simulink model "sim_models"  (R2018b)
settings: Solver=FixedStepAuto  StartTime=0.0  StopTime=10  RelTol=1e-3
values from neighbouring files (symbols this model uses):
  Ts = 0.1    [KinematicBicycleModel.m]    (also in LeftLaneChangeSinusoidalMotionModel.m; LinearizedBicycleModel.m; SimplifiedKinematicBicycleModel.m; amm_rel_test.m)
  vx = X(2)    [cv_model_fun.m]    (also in initialization.m = 10)
  vy = X(4)    [cv_model_fun.m]    (also in initialization.m = 0)
  x = X(1)    [KinematicBicycleModel.m]    (also in SimplifiedKinematicBicycleModel.m; behavior_model.m = 0:0.01:20; cca_model_fun.m; ctra_model_fun.m)
  y = X(2)    [KinematicBicycleModel.m]    (also in SimplifiedKinematicBicycleModel.m; behavior_model.m = [distances velocities]; cca_model_fun.m; ctra_model_fun.m)
libraries: simulink x1
settings Model: Creator=jasprit  LastModifiedBy=jasprit
settings SFSimCC: SimUseLocalCustomCode=off
settings RTWCC: RTWUseLocalCustomCode=off

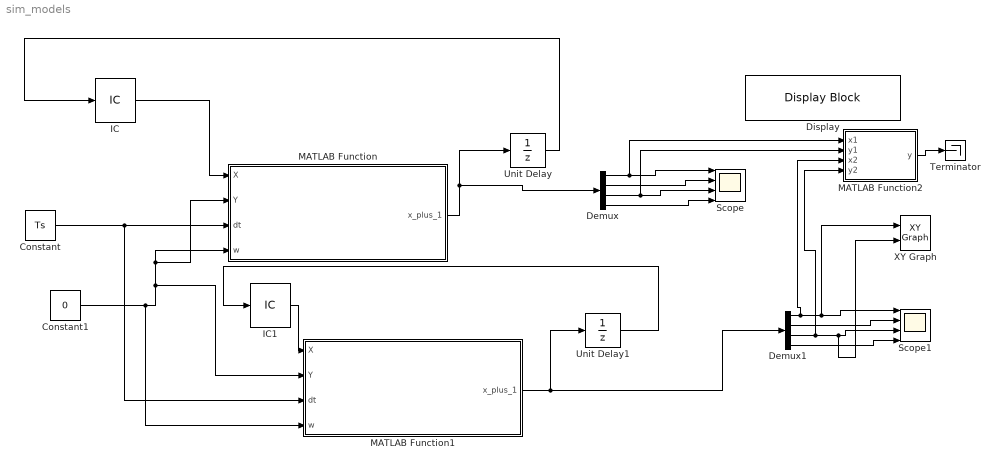
== system sim_models ==
  Constant : Constant  Value=Ts  SampleTime=Ts
  Constant1 : Constant  Value=0  SampleTime=Ts
  Demux : Demux
  Demux1 : Demux
  Display : DisplayBlock  WebBlockId=7  LabelPosition=Hide
  IC : InitialCondition  Value=[x vx y vy]
  IC1 : InitialCondition  Value=[50 0 50 -10]
  MATLAB Function : MATLAB Function  TreatAsAtomicUnit=on
  MATLAB Function1 : MATLAB Function  TreatAsAtomicUnit=on
  MATLAB Function2 : MATLAB Function  TreatAsAtomicUnit=on
  Scope : Scope  NumInputPorts=4
  Scope1 : Scope  NumInputPorts=4
  Terminator : Terminator
  Unit Delay : UnitDelay  SampleTime=-1
  Unit Delay1 : UnitDelay  SampleTime=-1
  XY Graph : simulink/Sinks/XY Graph  xmin=-10  xmax=200  ymin=-50  ymax=100  st=-1
  wires:
  MATLAB Function/1(x_plus_1) -> Demux/1, Unit Delay/1
  Constant/1 -> MATLAB Function1/3(dt), MATLAB Function/3(dt)
  Constant1/1 -> MATLAB Function1/4(w), MATLAB Function1/2(Y), MATLAB Function/2(Y), MATLAB Function/4(w)
  Unit Delay/1 -> IC/1
  Demux/1 -> MATLAB Function2/1(x1), Scope/1
  Demux/2 -> Scope/2
  Demux/3 -> MATLAB Function2/2(y1), Scope/3
  Demux/4 -> Scope/4
  IC/1 -> MATLAB Function/1(X)
  MATLAB Function1/1(x_plus_1) -> Demux1/1, Unit Delay1/1
  IC1/1 -> MATLAB Function1/1(X)
  Demux1/2 -> Scope1/2
  Unit Delay1/1 -> IC1/1
  Demux1/1 -> XY Graph/1, Scope1/1, MATLAB Function2/3(x2)
  Demux1/4 -> Scope1/4
  Demux1/3 -> MATLAB Function2/4(y2), XY Graph/2, Scope1/3
  MATLAB Function2/1(y) -> Terminator/1

== matlab function sim_models/MATLAB Function1 ==
  data: X input; x_plus_1 output; Y input; dt input; w input
function x_plus_1 = cv_model_fun(X, Y, dt, w)
    % X = [x vx y vy]'
    x_plus_1 = zeros(4,1)
    x = X(1);
    vx = X(2);
    y = X(3);
    vy = X(4);    
    x_plus_1 = [x + dt * vx; vx; y + dt * vy; vy];
end

== matlab function sim_models/MATLAB Function ==
  data: X input; x_plus_1 output; Y input; dt input; w input
function x_plus_1 = cv_model_fun(X, Y, dt, w)
    % X = [x vx y vy]'
%     x_plus_1 = zeros(4,1)
    x = X(1);
    vx = X(2);
    y = X(3);
    vy = X(4);    
    x_plus_1 = [x + dt * vx; vx; y + dt * vy; vy];
end

== matlab function sim_models/MATLAB Function2 ==
  data: x1 input; y output; y1 input; x2 input; y2 input
function y = fcn(x1, y1, x2, y2)
    coder.extrinsic('plot');
    
    x0 = [1:0.1:10];
    y0 = [11:0.1:20];
    x3 = [31:0.1:40];
    y3 = [41:0.1:50];
    plot(x0, y0, 'b', x3, y3, 'r');
%    legend('car1', 'car2');
    axis([-10 100 -10 100]);
    hold on
y = [x1 y1 x2 y2];
